simulink model "Ex9_2model"  (R2013a)
settings: Solver=ode45  StartTime=0.0  StopTime=1  RelTol=1e-3
settings Model: Creator=John  LastModifiedBy=John

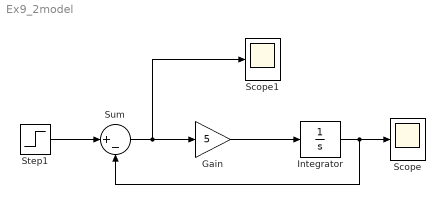
== system Ex9_2model ==
  Gain : Gain  Gain=5
  Integrator : Integrator
  Scope : Scope
  Scope1 : Scope
  Step1 : Step  Time=.01  SampleTime=0
  Sum : Sum  Inputs=|+-
  wires:
  Gain/1 -> Integrator/1
  Integrator/1 -> Sum/2, Scope/1
  Step1/1 -> Sum/1
  Sum/1 -> Scope1/1, Gain/1
